simulink model "untitled"  (R2020b)
settings: Solver=VariableStepAuto  StartTime=0.0  StopTime=1  RelTol=1e-3
settings Model: Creator=xpess  LastModifiedBy=xpess

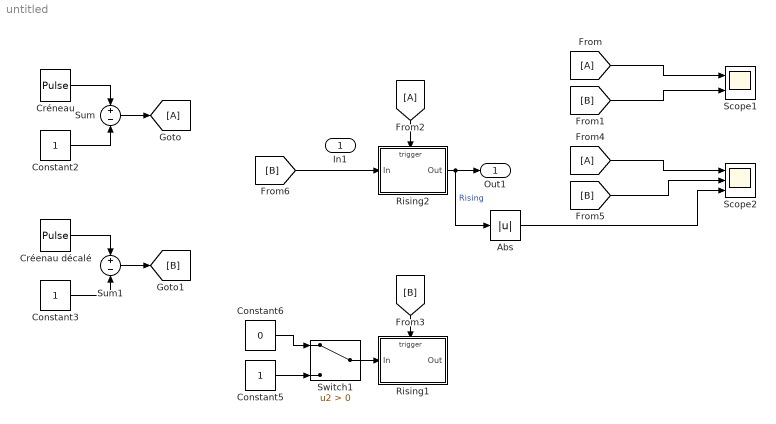
== system untitled ==
  In1 : Inport
  Abs : Abs
  Constant2 : Constant
  Constant3 : Constant
  Constant5 : Constant
  Constant6 : Constant  Value=0
  Créenau décalé : DiscretePulseGenerator  PulseType=Time based  Amplitude=2  Period=0.5  PulseWidth=50  PhaseDelay=0.5/4
  Créneau : DiscretePulseGenerator  PulseType=Time based  Amplitude=2  Period=0.5  PulseWidth=50
  Rising1 : Subsystem
  Rising2 : Subsystem
  Scope1 : Scope  NumInputPorts=2
  Scope2 : Scope  NumInputPorts=3
  Sum : Sum  Inputs=+|-
  Sum1 : Sum  Inputs=+|-
  Switch1 : Switch  Criteria=u2 > Threshold
  Out1 : Outport
  wires:
  Créneau/1 -> Sum/1
  Constant2/1 -> Sum/2
  Créenau décalé/1 -> Sum1/1
  Constant3/1 -> Sum1/2
  Sum/1 -> [A]
  Sum1/1 -> [B]
  [A] -> Scope1/1
  [B] -> Scope1/2
  [B] -> Rising2/1(In)
  [A] -> Rising2/Trigger
  [B] -> Rising1/Trigger
  Constant6/1 -> Switch1/1
  Constant5/1 -> Switch1/3
  Switch1/1 -> Rising1/1(In)
  Rising2/1(Out) -> Abs/1, Out1/1  "Rising"
  [B] -> Scope2/2
  [A] -> Scope2/1
  Abs/1 -> Scope2/3

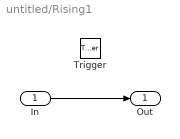
== system untitled/Rising1 ==
  In : Inport
  Trigger : TriggerPort  VariantControl=(inherit)
  Out : Outport  InitialOutput=0  VectorParamsAs1DForOutWhenUnconnected=off
  wires:
  In/1 -> Out/1

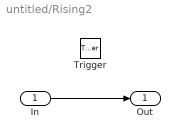
== system untitled/Rising2 ==
  In : Inport
  Trigger : TriggerPort  VariantControl=(inherit)
  Out : Outport  InitialOutput=0  VectorParamsAs1DForOutWhenUnconnected=off
  wires:
  In/1 -> Out/1
